simulink model "V2G_FDCC"  (R2024a)
settings: Solver=FixedStepAuto  StartTime=0.0  StopTime=10  FixedStep=1e-5  MaxStep=1.0E-5  RelTol=1e-3
values from neighbouring files (symbols this model uses):
  Batt_Ah = 2000    [main_v2gg2v.m]
  Batt_RespTime = 1    [main_v2gg2v.m]
  Batt_Vnom = 800    [main_v2gg2v.m]
  C_inv = (r*(Pinv/3)*al*(-be+al-1))/(100*Vac_l_rms*Vin_inv*wn*(al-be))    [main_v2gg2v.m]    (also in script.m = 0.00198943678865)
  C_mppt = 20*(Iout_mppt*D_mppt)/(deltaV*fs_mppt)    (= 0.0948148148148)    [main_v2gg2v.m]    (also in script.m)
  C_Vdc = 100*18e-3    (= 1.8)    [main_v2gg2v.m]
  cap_bat = 2000    [main_v2gg2v.m]    (also in script.m)
  Cbat_buck = deltaI_bat/(8*fs_bat*deltaV_bat)    (= 0.00133333333333)    [main_v2gg2v.m]    (also in script.m)
  Cdc = 30e-3    (= 0.03)    [main_v2gg2v.m]    (also in script.m)
  Cdc_boost = 50*Cbat_buck    (= 0.0666666666667)    [main_v2gg2v.m]    (also in script.m)
  Cf = 10*165e-6    (= 0.00165)    [main_v2gg2v.m]
  D = 2    [main_v2gg2v.m]
  Dinv = 0    [main_v2gg2v.m]
  f_grid = 50    [main_v2gg2v.m]
  fg = 50    [main_v2gg2v.m]    (also in script.m)
  H1 = 7    [main_v2gg2v.m]
  H2 = 8    [main_v2gg2v.m]
  H3 = 12    [main_v2gg2v.m]
  Hinv = 0    [main_v2gg2v.m]
  Ki_CC = 1    [main_v2gg2v.m]
  Ki_inner = 5000    [main_v2gg2v.m]
  Ki_outer = 10000    [main_v2gg2v.m]
  Ki_PLL = 10000    [main_v2gg2v.m]
  Kp_CC = 10    [main_v2gg2v.m]
  Kp_inner = 100    [main_v2gg2v.m]
  Kp_outer = 250    [main_v2gg2v.m]
  Kp_PLL = 100    [main_v2gg2v.m]
  L_bat = (Vbat*(Vdc_link-Vbat))/(deltaI_bat*fs_bat*Vdc_link)    (= 0.001875)    [main_v2gg2v.m]    (also in script.m)
  L_mppt = 1*(Vpv*D_mppt)/(deltaI*fs_mppt)    (= 0.000161333333333)    [main_v2gg2v.m]    (also in script.m)
  Lgrid = 1/10*0.69e-3    (= 6.9e-05)    [main_v2gg2v.m]
  Linv = 1/10*0.48e-3    (= 4.8e-05)    [main_v2gg2v.m]
  Lmin_inv = (100*Vac_l_rms*Vin_inv*(al-be))/(wn*r*(Pinv/3)*(-be+al-1))    [main_v2gg2v.m]    (also in script.m = 0.000611154981473)
  LowSat_CC = 0    [main_v2gg2v.m]
  omega = 2*pi*f_grid    (= 314.159265359)    [main_v2gg2v.m]
  Pinv = 2e6    (= 2000000)    [main_v2gg2v.m]    (also in script.m)
  Rd = 1.31    [main_v2gg2v.m]
  Sbase = 1e6    (= 1000000)    [main_v2gg2v.m]    (also in script.m)
  Snom_trafo = 1050e6    (= 1050000000)    [main_v2gg2v.m]
  t_fault_end = t_fault_start + FCT    (= 1.1)    [main_v2gg2v.m]
  t_fault_start = 1    [main_v2gg2v.m]
  Ts = 1e-5    (= 1e-05)    [main_v2gg2v.m]
  UpSat_CC = 1    [main_v2gg2v.m]
  Vac_inv = 800    [main_v2gg2v.m]    (also in script.m)
  Vbase = 345e3    (= 345000)    [main_v2gg2v.m]    (also in script.m)
  Vbat = 750    [main_v2gg2v.m]    (also in script.m)
  Vdc_ref = 1.5e3    (= 1500)    [main_v2gg2v.m]
  wg = 2*pi*fg    (= 314.159265359)    [main_v2gg2v.m]    (also in script.m)
undefined symbols (not defined in the file or in its folder): Acid, D1, Delta, h_PEV, Ibatfault_ref, ibatref, Ion, L12, L13, L23, Lbat, Lbuckboost, Lead, Lithium, R_Vdc, Rbuckboost, Vfault_thresh, vthref
libraries: spsSeriesRLCBranchLib x74, slpidlib x62, spsMosfetLib x50, spsGroundLib x48, spsBatteryLib x31, eeGeneralControl x31, spsPWMGeneratorDCDCLib x29, spsCurrentMeasurementLib x28, spsThreePhaseSeriesRLCBranchLib x21, spsThreePhaseVIMeasurementLib x18, spsIGBTDiodeLib x18, spsVoltageMeasurementLib x14
(part 1 of 11)
settings Model: Creator=BagaskaraPP  LastModifiedBy=hp
settings SolverCC: ZeroCrossAlgorithm=Adaptive  AlgebraicLoopSolver=TrustRegion
settings DataIOCC: ExternalInput=getinputstruct(op1)  InitialState=getstatestruct(op1)  SaveFormat=StructureWithTime  SaveOutput=off  ReturnWorkspaceOutputs=off  Refine=4
settings DebuggingCC: AlgebraicLoopMsg=none  MaxConsecutiveZCsMsg=none  IgnoredZcDiagnostic=none  ArithmeticOperatorsInVariantConditions=warning
settings ModelReferenceCC: EnableRefExpFcnMdlSchedulingChecks=on
settings SFSimCC: SimUseLocalCustomCode=off  CustomCodeUndefinedFunction=UseInterfaceOnly
settings RTWCC: RTWUseLocalCustomCode=off  GPUComputeCapability=3.5
settings CodeAppCC: StateflowObjectComments=on
settings SimscapeCC: SimscapeNormalizeSystem=off

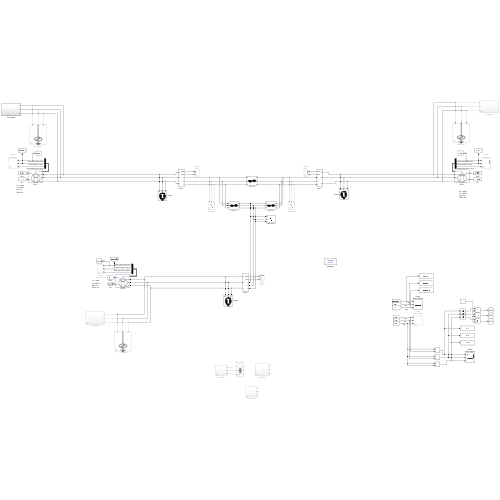
[thumbnail: Simulink's stored preview of the top-level diagram]
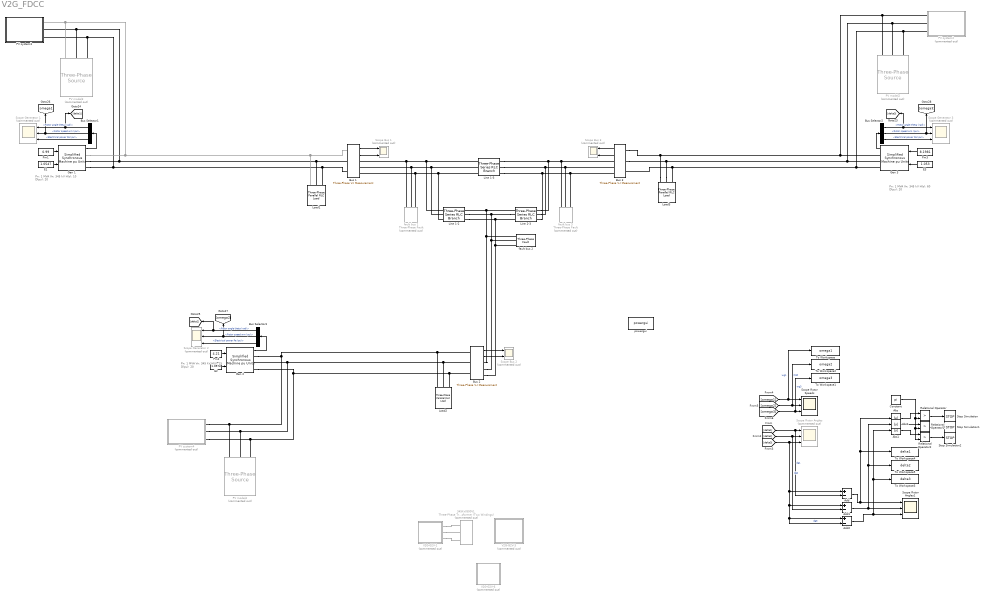
== system V2G_FDCC ==
  note: Pn: 1 MVA
      | Vn: 345 kV
      | H(s): 15
      | D(pu): 20
  note: Pn: 1 MVA
      | Vn: 345 kV
      | H(s): 60
      | D(pu): 20
  note: Pn: 1 MVA
      | Vn: 345 kV
      | H(s): 10
      | D(pu): 20
  345kV/800V1 : spsThreePhaseTransformerTwoWindingsLib/Three-Phase Transformer (Two Windings)  Commented=on  Winding1Connection=Delta (D1)  Winding2Connection=Yg  CoreType=Three single-phase transformers  SetSaturation=off  Hysteresis=off  DataFile='hysteresis'  SetInitialFlux=off  Measurements=None  UNITS=pu  NominalPower=[ Snom_trafo , f_grid ]  Winding1=[Vbase , 0 , 0 ]  Winding2=[ 800 , 0 , 0 ]  Rm=0  Lm=0  L0=0.5  Saturation=[ 0,0 ; 0.0024,1.2 ; 1.0,1.52 ]  InitialFluxes=[ 0.8 , -0.8 , 0.7 ]  BreakLoop=off  DiscreteSolver=Trapezoidal iterative  DataType=off  TransfoNumber=1
  Abs : Abs  SaturateOnIntegerOverflow=off
  Abs1 : Abs  SaturateOnIntegerOverflow=off
  Abs2 : Abs  SaturateOnIntegerOverflow=off
  Add : Sum  Inputs=+-
  Add1 : Sum  Inputs=+-
  Add2 : Sum  Inputs=+-
  Bus Selector1 : BusSelector  OutputSignals=Rotor angle theta (rad),Rotor speed wm (pu),Electrical power Pe (pu)
  Bus Selector2 : BusSelector  OutputSignals=Rotor angle theta (rad),Rotor speed wm (pu),Electrical power Pe (pu)
  Bus Selector3 : BusSelector  OutputSignals=Rotor angle theta (rad),Rotor speed wm (pu),Electrical power Pe (pu)
  Bus 1 : spsThreePhaseVIMeasurementLib/Three-Phase V-I Measurement  VoltageMeasurement=phase-to-ground  SetLabelV=off  LabelV=Vabc  Vpu=off  VpuLL=off  CurrentMeasurement=yes  SetLabelI=off  LabelI=Iabc  Ipu=off  Pbase=100e6  Vbase=500e3  OutputType=Complex  PhasorSimulation=off  PSBequivalent=0
  Bus 2 : spsThreePhaseVIMeasurementLib/Three-Phase V-I Measurement  VoltageMeasurement=phase-to-ground  SetLabelV=off  LabelV=Vabc  Vpu=off  VpuLL=off  CurrentMeasurement=yes  SetLabelI=off  LabelI=Iabc  Ipu=off  Pbase=100e6  Vbase=500e3  OutputType=Complex  PhasorSimulation=off  PSBequivalent=0
  Bus 3 : spsThreePhaseVIMeasurementLib/Three-Phase V-I Measurement  VoltageMeasurement=phase-to-ground  SetLabelV=off  LabelV=Vabc  Vpu=off  VpuLL=off  CurrentMeasurement=yes  SetLabelI=off  LabelI=Iabc  Ipu=off  Pbase=100e6  Vbase=500e3  OutputType=Complex  PhasorSimulation=off  PSBequivalent=0
  Constant : Constant  Value=pi
  E1 : Constant  Value=1.0547
  E2 : Constant  Value=1.0573
  E3 : Constant  Value=1.053
  Gen 1 : spsSimplifiedSynchronousMachinepuUnitsLib/Simplified Synchronous Machine pu Units  ConnectionType=3-wire Y  MechanicalLoad=Mechanical power Pm  MeasurementBus=off  NominalParameters=[Sbase Vbase f_grid]  Mechanical=[H1 D 1]  InternalRL="[0.0  0.088]"  InitialConditions=[0 19.7482 1.15593 1.15593 1.15593 -15.1433 -135.143 104.857]  IterativeDiscreteModel=Trapezoidal non iterative  TsBlock=-1  TsPowergui=0  LoadFlowParameters=[1,0,0,0,0]  Units=0  BusType=PV  Pref=1000000  Qref=0  Qmin=-Inf  Qmax=Inf  PLF=0  QLF=0
      settings: LibrarySourceBlock=|
      | sps_lib/Electrical Machines/Simplified Synchronous
      | Machine pu Units
  Gen 2 : spsSimplifiedSynchronousMachinepuUnitsLib/Simplified Synchronous Machine pu Units  ConnectionType=3-wire Y  MechanicalLoad=Mechanical power Pm  MeasurementBus=off  NominalParameters=[Sbase Vbase f_grid]  Mechanical=[H2 D 1]  InternalRL="[0.0  0.05]"  InitialConditions=[0 26.4733 4.27149 4.27149 4.27149 5.25563 -114.744 125.256]  IterativeDiscreteModel=Trapezoidal non iterative  TsBlock=-1  TsPowergui=0  LoadFlowParameters=[1,0,0,0,0]  Units=0  BusType=PV  Pref=4210000  Qref=0  Qmin=-Inf  Qmax=Inf  PLF=0  QLF=0
      settings: LibrarySourceBlock=|
      | sps_lib/Electrical Machines/Simplified Synchronous
      | Machine pu Units
  Gen 3 : spsSimplifiedSynchronousMachinepuUnitsLib/Simplified Synchronous Machine pu Units  ConnectionType=3-wire Y  MechanicalLoad=Mechanical power Pm  MeasurementBus=off  NominalParameters=[Sbase Vbase f_grid]  Mechanical=[H3 D 1]  InternalRL="[0.0  0.015]"  InitialConditions=[0 6.70648 8.74798 8.74798 8.74798 -20.4227 -140.423 99.5773]  IterativeDiscreteModel=Trapezoidal non iterative  TsBlock=-1  TsPowergui=0  LoadFlowParameters=[1,0,0,0,0]  Units=0  BusType=swing  Pref=6200000  Qref=0  Qmin=-Inf  Qmax=Inf  PLF=0  QLF=0
      settings: LibrarySourceBlock=|
      | sps_lib/Electrical Machines/Simplified Synchronous
      | Machine pu Units
  Line 1-2 : spsThreePhaseSeriesRLCBranchLib/Three-Phase Series RLC Branch  LConnTagsString=A|B|C  RConnTagsString=A|B|C  BranchType=RL  Resistance=0  Inductance=L12  Capacitance=1e-6  Measurements=None
  Line 1-3 : spsThreePhaseSeriesRLCBranchLib/Three-Phase Series RLC Branch  LConnTagsString=A|B|C  RConnTagsString=A|B|C  BranchType=RL  Resistance=0  Inductance=L13  Capacitance=1e-6  Measurements=None
  Line 2-3 : spsThreePhaseSeriesRLCBranchLib/Three-Phase Series RLC Branch  LConnTagsString=A|B|C  RConnTagsString=A|B|C  BranchType=RL  Resistance=0  Inductance=L23  Capacitance=1e-6  Measurements=None
  Load1 : spsThreePhaseParallelRLCLoadLib/Three-Phase Parallel RLC Load  LConnTagsString=A|B|C  Configuration=Y (grounded)  NominalVoltage=(345000)*1  Vabc=[1e3 1e3 1e3]  Vabcp=[1e3 1e3 1e3]  NominalFrequency=f_grid  UnbalancedPower=off  ActivePower=1500000  InductivePower=450000  CapacitivePower=0  Pabc=[10e3 9e3 11e3]  QLabc=[100 90 110]  QCabc=[100 90 110]  Pabcp=[10e3 9e3 11e3]  QLabcp=[100 90 110]  QCabcp=[100 90 110]  Measurements=None  LoadType=constant PQ
  Load2 : spsThreePhaseParallelRLCLoadLib/Three-Phase Parallel RLC Load  LConnTagsString=A|B|C  Configuration=Y (grounded)  NominalVoltage=(345000)*1  Vabc=[1e3 1e3 1e3]  Vabcp=[1e3 1e3 1e3]  NominalFrequency=f_grid  UnbalancedPower=off  ActivePower=1000000  InductivePower=300000  CapacitivePower=0  Pabc=[10e3 9e3 11e3]  QLabc=[100 90 110]  QCabc=[100 90 110]  Pabcp=[10e3 9e3 11e3]  QLabcp=[100 90 110]  QCabcp=[100 90 110]  Measurements=None  LoadType=constant PQ
  Load3 : spsThreePhaseParallelRLCLoadLib/Three-Phase Parallel RLC Load  LConnTagsString=A|B|C  Configuration=Y (grounded)  NominalVoltage=(345000)*1  Vabc=[1e3 1e3 1e3]  Vabcp=[1e3 1e3 1e3]  NominalFrequency=f_grid  UnbalancedPower=off  ActivePower=12400000  InductivePower=2500000  CapacitivePower=0  Pabc=[10e3 9e3 11e3]  QLabc=[100 90 110]  QCabc=[100 90 110]  Pabcp=[10e3 9e3 11e3]  QLabcp=[100 90 110]  QCabcp=[100 90 110]  Measurements=None  LoadType=constant PQ
  PV model2 : spsThreePhaseSourceLib/Three-Phase Source  Commented=on  InternalConnection=Yg  VoltagePhases=off  Voltage=(345000)*1  PhaseAngle=0  Voltage_phases=[25e3 25e3 25e3]/sqrt(3)  PhaseAngles_phases=[0 -120 +120]  Frequency=fg  NonIdealSource=off  SpecifyImpedance=off  Resistance=0.8929  Inductance=16.58e-3  ShortCircuitLevel=100e6  BaseVoltage=25e3  XRratio=7  BusType=PQ  Pref=1492000  Qref=606.9  Prefabc=[10e3, 10e3, 10e3]  Qrefabc=[0, 0, 0]  Qmin=-Inf  Qmax=Inf
  PV model3 : spsThreePhaseSourceLib/Three-Phase Source  Commented=on  InternalConnection=Yg  VoltagePhases=off  Voltage=(345000)*1  PhaseAngle=14.9621  Voltage_phases=[25e3 25e3 25e3]/sqrt(3)  PhaseAngles_phases=[0 -120 +120]  Frequency=fg  NonIdealSource=off  SpecifyImpedance=off  Resistance=0.8929  Inductance=16.58e-3  ShortCircuitLevel=100e6  BaseVoltage=25e3  XRratio=7  BusType=PQ  Pref=1492000  Qref=606.9  Prefabc=[10e3, 10e3, 10e3]  Qrefabc=[0, 0, 0]  Qmin=-Inf  Qmax=Inf
  PV model4 : spsThreePhaseSourceLib/Three-Phase Source  Commented=on  InternalConnection=Yg  VoltagePhases=off  Voltage=(345000)*1  PhaseAngle=21.4896  Voltage_phases=[25e3 25e3 25e3]/sqrt(3)  PhaseAngles_phases=[0 -120 +120]  Frequency=fg  NonIdealSource=off  SpecifyImpedance=off  Resistance=0.8929  Inductance=16.58e-3  ShortCircuitLevel=100e6  BaseVoltage=25e3  XRratio=7  BusType=PQ  Pref=1492000  Qref=606.9  Prefabc=[10e3, 10e3, 10e3]  Qrefabc=[0, 0, 0]  Qmin=-Inf  Qmax=Inf
  PV system2 : Subsystem  Commented=on
  PV system3 : Subsystem
  PV system4 : Subsystem  Commented=on
  Pm1 : Constant  Value=0.99
  Pm2 : Constant  Value=4.21
  Pm3 : Constant  Value=8.1981
  Relational Operator : RelationalOperator  Operator=>  OutDataTypeStr=boolean  RndMeth=Simplest  InputSameDT=off
  Relational Operator1 : RelationalOperator  Operator=>  OutDataTypeStr=boolean  RndMeth=Simplest  InputSameDT=off
  Relational Operator2 : RelationalOperator  Operator=>  OutDataTypeStr=boolean  RndMeth=Simplest  InputSameDT=off
  Scope Bus 1 : Scope  Commented=on  NumInputPorts=2
  Scope Bus 2 : Scope  Commented=on  NumInputPorts=2
  Scope Bus 3 : Scope  Commented=on  NumInputPorts=2
  Scope Generator 1 : Scope  Commented=on  NumInputPorts=3
  Scope Generator 2 : Scope  Commented=on  NumInputPorts=3
  Scope Generator 3 : Scope  Commented=on  NumInputPorts=3
  Scope Rotor Angles : Scope  Commented=on  NumInputPorts=3
  Scope Rotor Angles1 : Scope  NumInputPorts=3
  Scope Rotor Speeds : Scope  NumInputPorts=3
  Stop Simulation : Stop
  Stop Simulation1 : Stop
  Stop Simulation2 : Stop
  To Workspace : ToWorkspace  VariableName=omega1  SaveFormat=Timeseries  SampleTime=-1
  To Workspace1 : ToWorkspace  VariableName=omega3  SaveFormat=Timeseries  SampleTime=-1
  To Workspace2 : ToWorkspace  VariableName=omega2  SaveFormat=Timeseries  SampleTime=-1
  To Workspace3 : ToWorkspace  VariableName=delta3  SaveFormat=Timeseries  SampleTime=-1
  To Workspace4 : ToWorkspace  VariableName=delta1  SaveFormat=Timeseries  SampleTime=-1
  To Workspace5 : ToWorkspace  VariableName=delta2  SaveFormat=Timeseries  SampleTime=-1
  V2G-G2V-1 : Subsystem  Commented=on
  V2G-G2V-3 : Subsystem  Commented=on
  V2G-G2V-6 : Subsystem  Commented=on
  fault bus 1 : spsThreePhaseFaultLib/Three-Phase Fault  Commented=on  InitialStates=0  FaultA=on  FaultB=on  FaultC=on  GroundFault=off  SwitchTimes="[t_fault_start  t_fault_end]"  External=off  SwitchStatus=NaN  FaultResistance=0.001  GroundResistance=0.01  SnubberResistance=1e6  SnubberCapacitance=inf  Measurements=None
  fault bus 2 : spsThreePhaseFaultLib/Three-Phase Fault  InitialStates=0  FaultA=on  FaultB=on  FaultC=on  GroundFault=off  SwitchTimes="[t_fault_start  t_fault_end]"  External=off  SwitchStatus=NaN  FaultResistance=0.001  GroundResistance=0.01  SnubberResistance=1e6  SnubberCapacitance=inf  Measurements=None
  fault bus 3 : spsThreePhaseFaultLib/Three-Phase Fault  Commented=on  InitialStates=0  FaultA=on  FaultB=on  FaultC=on  GroundFault=off  SwitchTimes="[t_fault_start  t_fault_end]"  External=off  SwitchStatus=NaN  FaultResistance=0.001  GroundResistance=0.01  SnubberResistance=1e6  SnubberCapacitance=inf  Measurements=None
  powergui : sps_lib/powergui  Priority=1  SimulationMode=Discrete  SampleTime=1e-5  frequency=60  Iterations=200  frequencyindice=50  Pbase=1e6  ErrMax=1e-4  UnitsV=kV  UnitsW=MW  buscounter=1  FunctionMessages=off  echomessages=off  EnableUseOfTLC=off  CurrentSourceSwitches=off  DisableSnubberDevices=off  DisableRonSwitches=off  DisableVfSwitches=off  DisplayEquations=off  AutomaticDiscreteSolvers=off  SolverType=Tustin/Backward Euler (TBE)  Interpol=off  ExternalGateDelay=off  methode=off  Ts=100  x0status=blocks  SPID=on  SwTol=0  HookPort=off  NonlinearTolerance=1e-4  nMaxIteration=100  ContinueOnMaxIteration=off  RestoreLinks=warning  ResistiveCurrentMeasurement=off  Frange=[0:2:500]  Ylog=off  Xlog=on  ShowGrid=off  save=off  variable=ZData  structure=0  ZoomFFT=off  StartTime=0.0  cycles=1  DisplayStyle=1  fundamental=60  FreqAxis=off  MaxFrequency=1000  frequencyindicesteady=1  RmsSteady=1  display=off
  wires:
  Bus 1/1 -> Scope Bus 1/1
  Pm2/1 -> Gen 2/1
  Bus Selector2/2 -> [omega3], Scope Generator 3/2  "<Rotor speed wm (pu)>"
  Bus Selector2/1 -> Scope Generator 3/1, [delta3]  "<Rotor angle theta (rad)>"
  Pm3/1 -> Gen 3/1
  Bus 2/2 -> Scope Bus 2/2
  Bus Selector3/3 -> Scope Generator 2/3  "<Electrical power Pe (pu)>"
  Bus Selector2/3 -> Scope Generator 3/3  "<Electrical power Pe (pu)>"
  Bus 1/2 -> Scope Bus 1/2
  Bus Selector3/2 -> Scope Generator 2/2, [omega2]  "<Rotor speed wm (pu)>"
  Bus 3/2 -> Scope Bus 3/2
  Bus Selector3/1 -> Scope Generator 2/1, [delta2]  "<Rotor angle theta (rad)>"
  Bus 3/1 -> Scope Bus 3/1
  Bus 2/1 -> Scope Bus 2/1
  E1/1 -> Gen 1/2
  Pm1/1 -> Gen 1/1
  Gen 1/1 -> Bus Selector1/1
  Bus Selector1/3 -> Scope Generator 1/3  "<Electrical power Pe (pu)>"
  Gen 3/1 -> Bus Selector2/1
  Bus Selector1/2 -> Scope Generator 1/2, [omega1]  "<Rotor speed wm (pu)>"
  Bus Selector1/1 -> Scope Generator 1/1, [delta1]  "<Rotor angle theta (rad)>"
  Gen 2/1 -> Bus Selector3/1
  E2/1 -> Gen 2/2
  E3/1 -> Gen 3/2
  [omega2] -> To Workspace2/1, Scope Rotor Speeds/2  "wg2"
  [delta2] -> Add1/2, Scope Rotor Angles/2  "dg2"
  [delta3] -> Add/1, Add1/1, Add2/2, Add2/1, Scope Rotor Angles/3  "dg3"
  [delta1] -> Add/2, Scope Rotor Angles/1  "dg1"
  [omega3] -> To Workspace1/1, Scope Rotor Speeds/3  "wg3"
  [omega1] -> To Workspace/1, Scope Rotor Speeds/1  "wg1"
  Add1/1 -> Abs2/1, To Workspace5/1, Scope Rotor Angles1/2
  Add/1 -> Abs/1, To Workspace4/1, Scope Rotor Angles1/1
  Add2/1 -> Abs1/1, To Workspace3/1, Scope Rotor Angles1/3
  Abs/1 -> Relational Operator/1
  Abs2/1 -> Relational Operator1/1
  Abs1/1 -> Relational Operator2/1
  Relational Operator/1 -> Stop Simulation/1
  Constant/1 -> Relational Operator2/2, Relational Operator1/2, Relational Operator/2
  Relational Operator2/1 -> Stop Simulation2/1
  Relational Operator1/1 -> Stop Simulation1/1
  connections:
  Line 1-2/LConn1 -- Line 1-3/LConn1 -- fault bus 1/LConn1 -- Bus 1/RConn1
  Load1/LConn3 -- PV model3/RConn3 -- PV system3/RConn3 -- Gen 1/RConn3 -- Bus 1/LConn3
  Line 2-3/LConn2 -- Bus 2/RConn2 -- fault bus 2/LConn2 -- Line 1-2/RConn2
  Gen 3/RConn3 -- Bus 3/LConn3 -- Load3/LConn3 -- PV model2/RConn3 -- PV system2/RConn3
  Bus 3/RConn2 -- fault bus 3/LConn2 -- Line 2-3/RConn2 -- Line 1-3/RConn2
  Bus 3/RConn3 -- fault bus 3/LConn3 -- Line 2-3/RConn3 -- Line 1-3/RConn3
  PV system3/RConn2 -- PV model3/RConn2 -- Load1/LConn2 -- Bus 1/LConn2 -- Gen 1/RConn2
  Load3/LConn1 -- PV model2/RConn1 -- PV system2/RConn1 -- Gen 3/RConn1 -- Bus 3/LConn1
  Line 2-3/LConn1 -- Bus 2/RConn1 -- fault bus 2/LConn1 -- Line 1-2/RConn1
  Load3/LConn2 -- PV model2/RConn2 -- PV system2/RConn2 -- Gen 3/RConn2 -- Bus 3/LConn2
  Line 1-3/RConn1 -- Bus 3/RConn1 -- fault bus 3/LConn1 -- Line 2-3/RConn1
  Line 1-3/LConn2 -- Line 1-2/LConn2 -- fault bus 1/LConn2 -- Bus 1/RConn2
  Line 1-2/LConn3 -- Line 1-3/LConn3 -- fault bus 1/LConn3 -- Bus 1/RConn3
  PV model3/RConn1 -- PV system3/RConn1 -- Load1/LConn1 -- Bus 1/LConn1 -- Gen 1/RConn1
  Bus 2/RConn3 -- fault bus 2/LConn3 -- Line 2-3/LConn3 -- Line 1-2/RConn3
  V2G-G2V-1/LConn1 -- 345kV/800V1/RConn1
  V2G-G2V-1/LConn2 -- 345kV/800V1/RConn2
  V2G-G2V-1/LConn3 -- 345kV/800V1/RConn3
  Gen 2/RConn1 -- Load2/LConn1 -- Bus 2/LConn1 -- PV model4/RConn1 -- PV system4/RConn1
  Load2/LConn2 -- PV model4/RConn2 -- PV system4/RConn2 -- Gen 2/RConn2 -- Bus 2/LConn2
  Gen 2/RConn3 -- PV model4/RConn3 -- PV system4/RConn3 -- Bus 2/LConn3 -- Load2/LConn3

== system V2G_FDCC/PV system2 ==
  note: P = 1.96e6
      | Q = -0.6842
  Battery1 : spsBatteryLib/Battery  BatType=Lead-Acid  ShowTempParam=off  ThermalPreset="12.8V  40Ah  (LiFeMgPO4)"  ShowAgeParam=off  NomV=Vbat  NomQ=cap_bat  SOC=50  Batt_Tr=2  PresetModel=off  MaxQ=cap_bat  MinV=0.8*Vbat  FullV=1.1*Vbat  Dis_rate=Inom_bat  R=0.002  Normal_OP=0.9*cap_bat  expZone="[780   20]"  current=[250 500 750 1000]  Units=Ampere-hour  Tci=20  NomT=20  T2=-30  MaxQ2=4.8  FullV2=7.1  Normal_OP2=5.655  expZone2="[6.58           1]"  Rca=0.6  ti=2000  Dp=0  Neq0=0  Tsim=1e6  Ta1=25  Qeol=5.4*0.9  Reol=0.013333*1.2  Char_age=[2.3478, 3]  Dis_age=[2.3478, 10]  N1=1500  N2=10500  N3=1000  N4=1400  Ta2=45  N5=950
  Bus x : spsThreePhaseVIMeasurementLib/Three-Phase V-I Measurement  VoltageMeasurement=phase-to-ground  SetLabelV=off  LabelV=Vabc  Vpu=off  VpuLL=off  CurrentMeasurement=yes  SetLabelI=off  LabelI=Iabc  Ipu=off  Pbase=100e6  Vbase=13.8e3  OutputType=Complex  PhasorSimulation=off  PSBequivalent=0
  Cdc link1 : spsSeriesRLCBranchLib/Series RLC Branch  LConnTagsString=__new0  RConnTagsString=__new0  BranchType=C  Resistance=0.001  Inductance=1e-3  SetiL0=off  InitialCurrent=0  Capacitance=Cdc  Setx0=on  InitialVoltage=1500  Measurements=None
  Current Measurement1 : spsCurrentMeasurementLib/Current Measurement  PhasorSimulation=off  OutputType=Complex  PSBequivalent=0
  Current Measurement3 : spsCurrentMeasurementLib/Current Measurement  PhasorSimulation=off  OutputType=Complex  PSBequivalent=0
  DC-DC Converter Bidirectional1 : Subsystem
  DC-DC Converter Unidirectional1 : Subsystem
  Ground{2,9,12,14} (4 alike) : spsGroundLib/Ground  LConnTagsString=a
  Inverter : Subsystem
  Irradiance1 : Constant  Value=1000
  Ldc1 : spsSeriesRLCBranchLib/Series RLC Branch  LConnTagsString=__new0  RConnTagsString=__new0  BranchType=L  Resistance=0.002  Inductance=10e-3  SetiL0=off  InitialCurrent=0  Capacitance=5e-3  Setx0=on  InitialVoltage=0  Measurements=None
  Low-Pass Filter (Discrete or Continuous) : eeGeneralControl/Low-Pass Filter (Discrete or Continuous)  Commented=on  K=1  T=1/(2*pi*5)  B=inf  A=-inf  init_option=Inherited from block input  x0=0  Ts=-1
  Low-Pass Filter (Discrete or Continuous)2 : eeGeneralControl/Low-Pass Filter (Discrete or Continuous)  Commented=on  K=1  T=1/(2*pi*5)  B=inf  A=-inf  init_option=Inherited from block input  x0=0  Ts=-1
  PV Solar Array1 : spsPVArrayLib/PV Array  Npar=278  Nser=15  PlotType=array @ 1000 W/m2 & specified temperatures  S_vec=[ 1000 800 500 300 100 ]  Temp_C_vec=[ 20 25 30 35 ]  ModuleName=Sunpower SPR-X22-480-COM  PlotWhenSelected=off  Pm=480.32  Ncell=128  Voc=92.9  Isc=6.48  Vm=79  Im=6.08  beta_Voc_pc=-0.293  alpha_Isc_pc=0.031003  beta_Voc=-0.2722  alpha_Isc=0.002009  IL=6.4884  I0=1.5908e-11  nI=1.0576  Rsh=598.2816  Rs=0.48607  RobustModel=off  RobustCellTemperature=313.3991  BAL=on  Tc=1e-6  Tfilter=5e-5
  PV model2 : spsThreePhaseSourceLib/Three-Phase Source  Commented=on  InternalConnection=Yg  VoltagePhases=off  Voltage=(345000)*1  PhaseAngle=0  Voltage_phases=[25e3 25e3 25e3]/sqrt(3)  PhaseAngles_phases=[0 -120 +120]  Frequency=fg  NonIdealSource=off  SpecifyImpedance=off  Resistance=0.8929  Inductance=16.58e-3  ShortCircuitLevel=100e6  BaseVoltage=25e3  XRratio=7  BusType=swing  Pref=1993000  Qref=10680  Prefabc=[10e3, 10e3, 10e3]  Qrefabc=[0, 0, 0]  Qmin=-Inf  Qmax=Inf
  Power (Positive-Sequence) : spsPowerPositiveSequenceLib/Power (Positive-Sequence)  Commented=on  Freq=50  Vinit=[0, 0]  Iinit=[0, 0]  Ts=1e-5
      settings: LibrarySourceBlock=|
      | sps_lib/Sensors and Measurements/Power
      | (Positive-Sequence)
  Product : Product  Commented=on
  Scope3 : Scope  Commented=on  NumInputPorts=2
  Scope5 : Scope  Commented=on  NumInputPorts=2
  Scope9 : Scope  Commented=on  NumInputPorts=3
  Temp1 : Constant  Value=25
  Three-Phase Transformer : spsThreePhaseTransformerTwoWindingsLib/Three-Phase Transformer (Two Windings)  Winding1Connection=Yg  Winding2Connection=Delta (D1)  CoreType=Three single-phase transformers  SetSaturation=off  Hysteresis=off  DataFile='hysteresis'  SetInitialFlux=off  Measurements=None  UNITS=pu  NominalPower=[ Pinv*2 , fg ]  Winding1=[Vbase 1e-6 1e-6]  Winding2=[Vac_inv 1e-6 1e-6]  Rm=500  Lm=1000  L0=0.5  Saturation=[0 0;0.01 0.9;0.05 1]  InitialFluxes=[-1.0025142026259 0.501432695325379 0.501081507300505]  BreakLoop=off  DiscreteSolver=Trapezoidal iterative  DataType=off  TransfoNumber=1
  Voltage Measurement1 : spsVoltageMeasurementLib/Voltage Measurement  PhasorSimulation=off  OutputType=Complex  PSBequivalent=0
  Voltage Measurement2 : spsVoltageMeasurementLib/Voltage Measurement  PhasorSimulation=off  OutputType=Complex  PSBequivalent=0
  a : PMIOPort  Side=Right
  b : PMIOPort  Port=2  Side=Right
  c : PMIOPort  Port=3  Side=Right
  wires:
  Voltage Measurement2/1 -> Scope5/1  "Vout"
  Irradiance1/1 -> PV Solar Array1/1
  Low-Pass Filter (Discrete or Continuous)/1 -> Scope3/1  "Pout"
  Power (Positive-Sequence)/1 -> Low-Pass Filter (Discrete or Continuous)/1
  Current Measurement1/1 -> Scope5/2  "iout"
  Voltage Measurement1/1 -> [Vdc], Product/1, Scope9/1
  Current Measurement3/1 -> Product/2, Scope9/2
  Low-Pass Filter (Discrete or Continuous)2/1 -> Scope3/2  "Qout"
  [Vdc] -> DC-DC Converter Bidirectional1/1(Vdclink)
  Bus x/2 -> Power (Positive-Sequence)/2
  Temp1/1 -> PV Solar Array1/2
  Bus x/1 -> Power (Positive-Sequence)/1
  Power (Positive-Sequence)/2 -> Low-Pass Filter (Discrete or Continuous)2/1
  Product/1 -> Scope9/3
  connections:
  Inverter/RConn1 -- Current Measurement1/LConn1
  PV Solar Array1/RConn1 -- DC-DC Converter Unidirectional1/LConn1
  Voltage Measurement2/LConn1 -- Current Measurement1/RConn1 -- Three-Phase Transformer/RConn1
  Voltage Measurement2/LConn2 -- Inverter/RConn2 -- Three-Phase Transformer/RConn2
  Inverter/LConn1 -- Voltage Measurement1/LConn1 -- Current Measurement3/RConn1
  Three-Phase Transformer/RConn3 -- Inverter/RConn3
  Battery1/LConn2 -- Ground2/LConn1
  Three-Phase Transformer/LConn3 -- Bus x/LConn3
  Voltage Measurement1/LConn2 -- Ground9/LConn1
  PV Solar Array1/RConn2 -- Ground14/LConn1
  Battery1/LConn1 -- DC-DC Converter Bidirectional1/LConn1
  Ground12/LConn1 -- Cdc link1/RConn1
  Three-Phase Transformer/LConn1 -- Bus x/LConn1
  Current Measurement3/LConn1 -- Cdc link1/LConn1 -- DC-DC Converter Bidirectional1/RConn1 -- Ldc1/RConn1
  Three-Phase Transformer/LConn2 -- Bus x/LConn2
  Ldc1/LConn1 -- DC-DC Converter Unidirectional1/RConn1
  Bus x/RConn2 -- b/RConn1 -- PV model2/RConn2
  Bus x/RConn1 -- a/RConn1 -- PV model2/RConn1
  Bus x/RConn3 -- c/RConn1 -- PV model2/RConn3

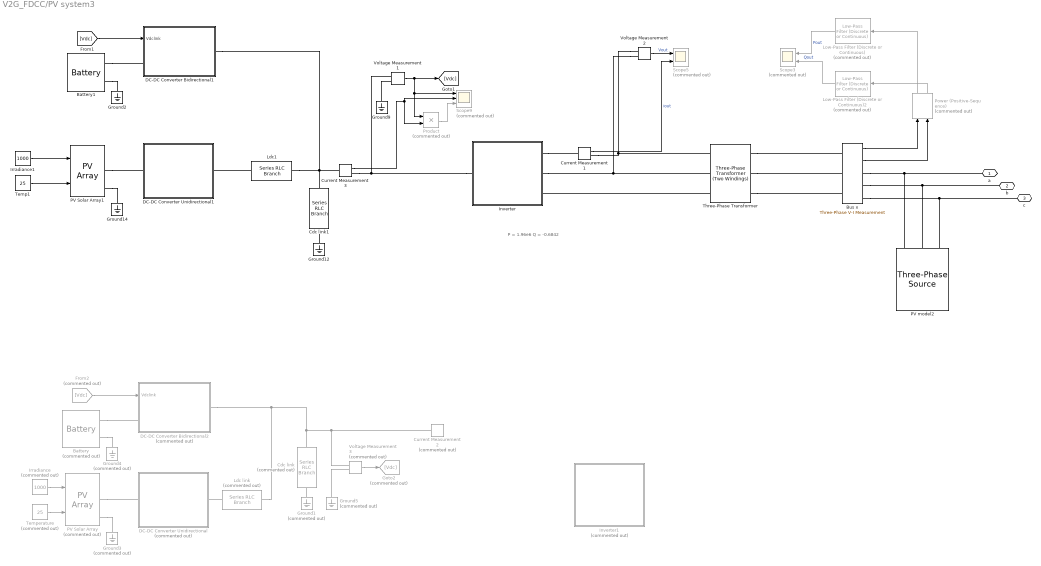
== system V2G_FDCC/PV system3 ==
  note: P = 1.96e6
      | Q = -0.6842
  Battery : spsBatteryLib/Battery  Commented=on  BatType=Lead-Acid  ShowTempParam=off  ThermalPreset="12.8V  40Ah  (LiFeMgPO4)"  ShowAgeParam=off  NomV=Vbat  NomQ=cap_bat  SOC=50  Batt_Tr=2  PresetModel=off  MaxQ=cap_bat  MinV=0.8*Vbat  FullV=1.1*Vbat  Dis_rate=Inom_bat  R=0.002  Normal_OP=0.9*cap_bat  expZone="[780   20]"  current=[250 500 750 1000]  Units=Ampere-hour  Tci=20  NomT=20  T2=-30  MaxQ2=4.8  FullV2=7.1  Normal_OP2=5.655  expZone2="[6.58           1]"  Rca=0.6  ti=2000  Dp=0  Neq0=0  Tsim=1e6  Ta1=25  Qeol=5.4*0.9  Reol=0.013333*1.2  Char_age=[2.3478, 3]  Dis_age=[2.3478, 10]  N1=1500  N2=10500  N3=1000  N4=1400  Ta2=45  N5=950
  Battery1 : spsBatteryLib/Battery  BatType=Lead-Acid  ShowTempParam=off  ThermalPreset="12.8V  40Ah  (LiFeMgPO4)"  ShowAgeParam=off  NomV=Vbat  NomQ=cap_bat  SOC=50  Batt_Tr=2  PresetModel=off  MaxQ=cap_bat  MinV=0.8*Vbat  FullV=1.1*Vbat  Dis_rate=Inom_bat  R=0.002  Normal_OP=0.9*cap_bat  expZone="[780   20]"  current=[250 500 750 1000]  Units=Ampere-hour  Tci=20  NomT=20  T2=-30  MaxQ2=4.8  FullV2=7.1  Normal_OP2=5.655  expZone2="[6.58           1]"  Rca=0.6  ti=2000  Dp=0  Neq0=0  Tsim=1e6  Ta1=25  Qeol=5.4*0.9  Reol=0.013333*1.2  Char_age=[2.3478, 3]  Dis_age=[2.3478, 10]  N1=1500  N2=10500  N3=1000  N4=1400  Ta2=45  N5=950
  Bus x : spsThreePhaseVIMeasurementLib/Three-Phase V-I Measurement  VoltageMeasurement=phase-to-ground  SetLabelV=off  LabelV=Vabc  Vpu=off  VpuLL=off  CurrentMeasurement=yes  SetLabelI=off  LabelI=Iabc  Ipu=off  Pbase=100e6  Vbase=13.8e3  OutputType=Complex  PhasorSimulation=off  PSBequivalent=0
  Cdc link : spsSeriesRLCBranchLib/Series RLC Branch  Commented=on  LConnTagsString=__new0  RConnTagsString=__new0  BranchType=C  Resistance=0.001  Inductance=1e-3  SetiL0=off  InitialCurrent=0  Capacitance=Cdc  Setx0=on  InitialVoltage=1500  Measurements=None
  Cdc link1 : spsSeriesRLCBranchLib/Series RLC Branch  LConnTagsString=__new0  RConnTagsString=__new0  BranchType=C  Resistance=0.001  Inductance=1e-3  SetiL0=off  InitialCurrent=0  Capacitance=Cdc  Setx0=on  InitialVoltage=1500  Measurements=None
  Current Measurement1 : spsCurrentMeasurementLib/Current Measurement  PhasorSimulation=off  OutputType=Complex  PSBequivalent=0
  Current Measurement2 : spsCurrentMeasurementLib/Current Measurement  Commented=on  PhasorSimulation=off  OutputType=Complex  PSBequivalent=0
  Current Measurement3 : spsCurrentMeasurementLib/Current Measurement  PhasorSimulation=off  OutputType=Complex  PSBequivalent=0
  DC-DC Converter Bidirectional1 : Subsystem
  DC-DC Converter Bidirectional2 : Subsystem  Commented=on
  DC-DC Converter Unidirectional : Subsystem  Commented=on
  DC-DC Converter Unidirectional1 : Subsystem
  From2 : From  Commented=on  GotoTag=Vdc
  Goto2 : Goto  Commented=on  GotoTag=Vdc
  Ground{1,3..5} (4 alike) : spsGroundLib/Ground  Commented=on  LConnTagsString=a
  Ground{2,9,12,14} (4 alike) : spsGroundLib/Ground  LConnTagsString=a
  Inverter : Subsystem
  Inverter1 : Subsystem  Commented=on
  Irradiance : Constant  Commented=on  Value=1000
  Irradiance1 : Constant  Value=1000
  Ldc link : spsSeriesRLCBranchLib/Series RLC Branch  Commented=on  LConnTagsString=__new0  RConnTagsString=__new0  BranchType=L  Resistance=0.002  Inductance=10e-3  SetiL0=off  InitialCurrent=0  Capacitance=5e-3  Setx0=on  InitialVoltage=0  Measurements=None
  Ldc1 : spsSeriesRLCBranchLib/Series RLC Branch  LConnTagsString=__new0  RConnTagsString=__new0  BranchType=L  Resistance=0.002  Inductance=10e-3  SetiL0=off  InitialCurrent=0  Capacitance=5e-3  Setx0=on  InitialVoltage=0  Measurements=None
  Low-Pass Filter (Discrete or Continuous) : eeGeneralControl/Low-Pass Filter (Discrete or Continuous)  Commented=on  K=1  T=1/(2*pi*5)  B=inf  A=-inf  init_option=Inherited from block input  x0=0  Ts=-1
  Low-Pass Filter (Discrete or Continuous)2 : eeGeneralControl/Low-Pass Filter (Discrete or Continuous)  Commented=on  K=1  T=1/(2*pi*5)  B=inf  A=-inf  init_option=Inherited from block input  x0=0  Ts=-1
  PV Solar Array : spsPVArrayLib/PV Array  Commented=on  Npar=278  Nser=15  PlotType=array @ 1000 W/m2 & specified temperatures  S_vec=[ 1000 800 500 300 100 ]  Temp_C_vec=[ 20 25 30 35 ]  ModuleName=Sunpower SPR-X22-480-COM  PlotWhenSelected=off  Pm=480.32  Ncell=128  Voc=92.9  Isc=6.48  Vm=79  Im=6.08  beta_Voc_pc=-0.293  alpha_Isc_pc=0.031003  beta_Voc=-0.2722  alpha_Isc=0.002009  IL=6.4884  I0=1.5908e-11  nI=1.0576  Rsh=598.2816  Rs=0.48607  RobustModel=off  RobustCellTemperature=313.3991  BAL=on  Tc=1e-6  Tfilter=5e-5
  PV Solar Array1 : spsPVArrayLib/PV Array  Npar=278  Nser=15  PlotType=array @ 1000 W/m2 & specified temperatures  S_vec=[ 1000 800 500 300 100 ]  Temp_C_vec=[ 20 25 30 35 ]  ModuleName=Sunpower SPR-X22-480-COM  PlotWhenSelected=off  Pm=480.32  Ncell=128  Voc=92.9  Isc=6.48  Vm=79  Im=6.08  beta_Voc_pc=-0.293  alpha_Isc_pc=0.031003  beta_Voc=-0.2722  alpha_Isc=0.002009  IL=6.4884  I0=1.5908e-11  nI=1.0576  Rsh=598.2816  Rs=0.48607  RobustModel=off  RobustCellTemperature=313.3991  BAL=on  Tc=1e-6  Tfilter=5e-5
  PV model2 : spsThreePhaseSourceLib/Three-Phase Source  InternalConnection=Yg  VoltagePhases=off  Voltage=(345000)*1  PhaseAngle=0  Voltage_phases=[25e3 25e3 25e3]/sqrt(3)  PhaseAngles_phases=[0 -120 +120]  Frequency=fg  NonIdealSource=off  SpecifyImpedance=off  Resistance=0.8929  Inductance=16.58e-3  ShortCircuitLevel=100e6  BaseVoltage=25e3  XRratio=7  BusType=swing  Pref=1993000  Qref=10680  Prefabc=[10e3, 10e3, 10e3]  Qrefabc=[0, 0, 0]  Qmin=-Inf  Qmax=Inf
  Power (Positive-Sequence) : spsPowerPositiveSequenceLib/Power (Positive-Sequence)  Commented=on  Freq=50  Vinit=[0, 0]  Iinit=[0, 0]  Ts=1e-5
      settings: LibrarySourceBlock=|
      | sps_lib/Sensors and Measurements/Power
      | (Positive-Sequence)
  Product : Product  Commented=on
  Scope3 : Scope  Commented=on  NumInputPorts=2
  Scope5 : Scope  Commented=on  NumInputPorts=2
  Scope9 : Scope  Commented=on  NumInputPorts=3
  Temp1 : Constant  Value=25
  Temperature : Constant  Commented=on  Value=25
  Three-Phase Transformer : spsThreePhaseTransformerTwoWindingsLib/Three-Phase Transformer (Two Windings)  Winding1Connection=Yg  Winding2Connection=Delta (D1)  CoreType=Three single-phase transformers  SetSaturation=off  Hysteresis=off  DataFile='hysteresis'  SetInitialFlux=off  Measurements=None  UNITS=pu  NominalPower=[ Pinv*2 , fg ]  Winding1=[Vbase 1e-6 1e-6]  Winding2=[Vac_inv 1e-6 1e-6]  Rm=500  Lm=1000  L0=0.5  Saturation=[0 0;0.01 0.9;0.05 1]  InitialFluxes=[-1.0025142026259 0.501432695325379 0.501081507300505]  BreakLoop=off  DiscreteSolver=Trapezoidal iterative  DataType=off  TransfoNumber=1
  Voltage Measurement1 : spsVoltageMeasurementLib/Voltage Measurement  PhasorSimulation=off  OutputType=Complex  PSBequivalent=0
  Voltage Measurement2 : spsVoltageMeasurementLib/Voltage Measurement  PhasorSimulation=off  OutputType=Complex  PSBequivalent=0
  Voltage Measurement3 : spsVoltageMeasurementLib/Voltage Measurement  Commented=on  PhasorSimulation=off  OutputType=Complex  PSBequivalent=0
  a : PMIOPort  Side=Right
  b : PMIOPort  Port=2  Side=Right
  c : PMIOPort  Port=3  Side=Right
  wires:
  Voltage Measurement2/1 -> Scope5/1  "Vout"
  Irradiance1/1 -> PV Solar Array1/1
  Low-Pass Filter (Discrete or Continuous)/1 -> Scope3/1  "Pout"
  Power (Positive-Sequence)/1 -> Low-Pass Filter (Discrete or Continuous)/1
  Current Measurement1/1 -> Scope5/2  "iout"
  Voltage Measurement1/1 -> [Vdc], Product/1, Scope9/1
  Current Measurement3/1 -> Product/2, Scope9/2
  Low-Pass Filter (Discrete or Continuous)2/1 -> Scope3/2  "Qout"
  [Vdc] -> DC-DC Converter Bidirectional1/1(Vdclink)
  Bus x/2 -> Power (Positive-Sequence)/2
  Temp1/1 -> PV Solar Array1/2
  Bus x/1 -> Power (Positive-Sequence)/1
  Power (Positive-Sequence)/2 -> Low-Pass Filter (Discrete or Continuous)2/1
  Product/1 -> Scope9/3
  Temperature/1 -> PV Solar Array/2
  Voltage Measurement3/1 -> Goto2/1
  From2/1 -> DC-DC Converter Bidirectional2/1(Vdclink)
  Irradiance/1 -> PV Solar Array/1
  connections:
  Inverter/RConn1 -- Current Measurement1/LConn1
  PV Solar Array1/RConn1 -- DC-DC Converter Unidirectional1/LConn1
  Voltage Measurement2/LConn1 -- Current Measurement1/RConn1 -- Three-Phase Transformer/RConn1
  Voltage Measurement2/LConn2 -- Inverter/RConn2 -- Three-Phase Transformer/RConn2
  Inverter/LConn1 -- Voltage Measurement1/LConn1 -- Current Measurement3/RConn1
  Three-Phase Transformer/RConn3 -- Inverter/RConn3
  Battery1/LConn2 -- Ground2/LConn1
  Three-Phase Transformer/LConn3 -- Bus x/LConn3
  Voltage Measurement1/LConn2 -- Ground9/LConn1
  PV Solar Array1/RConn2 -- Ground14/LConn1
  Battery1/LConn1 -- DC-DC Converter Bidirectional1/LConn1
  Ground12/LConn1 -- Cdc link1/RConn1
  Three-Phase Transformer/LConn1 -- Bus x/LConn1
  Current Measurement3/LConn1 -- Cdc link1/LConn1 -- DC-DC Converter Bidirectional1/RConn1 -- Ldc1/RConn1
  Three-Phase Transformer/LConn2 -- Bus x/LConn2
  Ldc1/LConn1 -- DC-DC Converter Unidirectional1/RConn1
  Bus x/RConn2 -- b/RConn1 -- PV model2/RConn2
  Bus x/RConn1 -- a/RConn1 -- PV model2/RConn1
  Bus x/RConn3 -- c/RConn1 -- PV model2/RConn3
  Ldc link/RConn1 -- Cdc link/LConn1 -- Current Measurement2/LConn1 -- Voltage Measurement3/LConn1 -- DC-DC Converter Bidirectional2/RConn1
  Ldc link/LConn1 -- DC-DC Converter Unidirectional/RConn1
  PV Solar Array/RConn1 -- DC-DC Converter Unidirectional/LConn1
  PV Solar Array/RConn2 -- Ground3/LConn1
  Voltage Measurement3/LConn2 -- Ground5/LConn1
  Ground1/LConn1 -- Cdc link/RConn1
  Battery/LConn2 -- Ground4/LConn1
  Battery/LConn1 -- DC-DC Converter Bidirectional2/LConn1

== system V2G_FDCC/PV system4 ==
  note: P = 1.96e6
      | Q = -0.6842
  Battery1 : spsBatteryLib/Battery  BatType=Lead-Acid  ShowTempParam=off  ThermalPreset="12.8V  40Ah  (LiFeMgPO4)"  ShowAgeParam=off  NomV=Vbat  NomQ=cap_bat  SOC=50  Batt_Tr=2  PresetModel=off  MaxQ=cap_bat  MinV=0.8*Vbat  FullV=1.1*Vbat  Dis_rate=Inom_bat  R=0.002  Normal_OP=0.9*cap_bat  expZone="[780   20]"  current=[250 500 750 1000]  Units=Ampere-hour  Tci=20  NomT=20  T2=-30  MaxQ2=4.8  FullV2=7.1  Normal_OP2=5.655  expZone2="[6.58           1]"  Rca=0.6  ti=2000  Dp=0  Neq0=0  Tsim=1e6  Ta1=25  Qeol=5.4*0.9  Reol=0.013333*1.2  Char_age=[2.3478, 3]  Dis_age=[2.3478, 10]  N1=1500  N2=10500  N3=1000  N4=1400  Ta2=45  N5=950
  Bus x : spsThreePhaseVIMeasurementLib/Three-Phase V-I Measurement  VoltageMeasurement=phase-to-ground  SetLabelV=off  LabelV=Vabc  Vpu=off  VpuLL=off  CurrentMeasurement=yes  SetLabelI=off  LabelI=Iabc  Ipu=off  Pbase=100e6  Vbase=13.8e3  OutputType=Complex  PhasorSimulation=off  PSBequivalent=0
  Cdc link1 : spsSeriesRLCBranchLib/Series RLC Branch  LConnTagsString=__new0  RConnTagsString=__new0  BranchType=C  Resistance=0.001  Inductance=1e-3  SetiL0=off  InitialCurrent=0  Capacitance=Cdc  Setx0=on  InitialVoltage=1500  Measurements=None
  Current Measurement1 : spsCurrentMeasurementLib/Current Measurement  PhasorSimulation=off  OutputType=Complex  PSBequivalent=0
  Current Measurement3 : spsCurrentMeasurementLib/Current Measurement  PhasorSimulation=off  OutputType=Complex  PSBequivalent=0
  DC-DC Converter Bidirectional1 : Subsystem
  DC-DC Converter Unidirectional1 : Subsystem
  Ground{2,9,12,14} (4 alike) : spsGroundLib/Ground  LConnTagsString=a
  Inverter : Subsystem
  Irradiance1 : Constant  Value=1000
  Ldc1 : spsSeriesRLCBranchLib/Series RLC Branch  LConnTagsString=__new0  RConnTagsString=__new0  BranchType=L  Resistance=0.002  Inductance=10e-3  SetiL0=off  InitialCurrent=0  Capacitance=5e-3  Setx0=on  InitialVoltage=0  Measurements=None
  Low-Pass Filter (Discrete or Continuous) : eeGeneralControl/Low-Pass Filter (Discrete or Continuous)  Commented=on  K=1  T=1/(2*pi*5)  B=inf  A=-inf  init_option=Inherited from block input  x0=0  Ts=-1
  Low-Pass Filter (Discrete or Continuous)2 : eeGeneralControl/Low-Pass Filter (Discrete or Continuous)  Commented=on  K=1  T=1/(2*pi*5)  B=inf  A=-inf  init_option=Inherited from block input  x0=0  Ts=-1
  PV Solar Array1 : spsPVArrayLib/PV Array  Npar=278  Nser=15  PlotType=array @ 1000 W/m2 & specified temperatures  S_vec=[ 1000 800 500 300 100 ]  Temp_C_vec=[ 20 25 30 35 ]  ModuleName=Sunpower SPR-X22-480-COM  PlotWhenSelected=off  Pm=480.32  Ncell=128  Voc=92.9  Isc=6.48  Vm=79  Im=6.08  beta_Voc_pc=-0.293  alpha_Isc_pc=0.031003  beta_Voc=-0.2722  alpha_Isc=0.002009  IL=6.4884  I0=1.5908e-11  nI=1.0576  Rsh=598.2816  Rs=0.48607  RobustModel=off  RobustCellTemperature=313.3991  BAL=on  Tc=1e-6  Tfilter=5e-5
  PV model2 : spsThreePhaseSourceLib/Three-Phase Source  Commented=on  InternalConnection=Yg  VoltagePhases=off  Voltage=(345000)*1  PhaseAngle=0  Voltage_phases=[25e3 25e3 25e3]/sqrt(3)  PhaseAngles_phases=[0 -120 +120]  Frequency=fg  NonIdealSource=off  SpecifyImpedance=off  Resistance=0.8929  Inductance=16.58e-3  ShortCircuitLevel=100e6  BaseVoltage=25e3  XRratio=7  BusType=swing  Pref=1993000  Qref=10680  Prefabc=[10e3, 10e3, 10e3]  Qrefabc=[0, 0, 0]  Qmin=-Inf  Qmax=Inf
  Power (Positive-Sequence) : spsPowerPositiveSequenceLib/Power (Positive-Sequence)  Commented=on  Freq=50  Vinit=[0, 0]  Iinit=[0, 0]  Ts=1e-5
      settings: LibrarySourceBlock=|
      | sps_lib/Sensors and Measurements/Power
      | (Positive-Sequence)
  Product : Product  Commented=on
  Scope3 : Scope  Commented=on  NumInputPorts=2
  Scope5 : Scope  Commented=on  NumInputPorts=2
  Scope9 : Scope  Commented=on  NumInputPorts=3
  Temp1 : Constant  Value=25
  Three-Phase Transformer : spsThreePhaseTransformerTwoWindingsLib/Three-Phase Transformer (Two Windings)  Winding1Connection=Yg  Winding2Connection=Delta (D1)  CoreType=Three single-phase transformers  SetSaturation=off  Hysteresis=off  DataFile='hysteresis'  SetInitialFlux=off  Measurements=None  UNITS=pu  NominalPower=[ Pinv*2 , fg ]  Winding1=[Vbase 1e-6 1e-6]  Winding2=[Vac_inv 1e-6 1e-6]  Rm=500  Lm=1000  L0=0.5  Saturation=[0 0;0.01 0.9;0.05 1]  InitialFluxes=[-1.0025142026259 0.501432695325379 0.501081507300505]  BreakLoop=off  DiscreteSolver=Trapezoidal iterative  DataType=off  TransfoNumber=1
  Voltage Measurement1 : spsVoltageMeasurementLib/Voltage Measurement  PhasorSimulation=off  OutputType=Complex  PSBequivalent=0
  Voltage Measurement2 : spsVoltageMeasurementLib/Voltage Measurement  PhasorSimulation=off  OutputType=Complex  PSBequivalent=0
  a : PMIOPort  Side=Right
  b : PMIOPort  Port=2  Side=Right
  c : PMIOPort  Port=3  Side=Right
  wires:
  Voltage Measurement2/1 -> Scope5/1  "Vout"
  Irradiance1/1 -> PV Solar Array1/1
  Low-Pass Filter (Discrete or Continuous)/1 -> Scope3/1  "Pout"
  Power (Positive-Sequence)/1 -> Low-Pass Filter (Discrete or Continuous)/1
  Current Measurement1/1 -> Scope5/2  "iout"
  Voltage Measurement1/1 -> [Vdc], Product/1, Scope9/1
  Current Measurement3/1 -> Product/2, Scope9/2
  Low-Pass Filter (Discrete or Continuous)2/1 -> Scope3/2  "Qout"
  [Vdc] -> DC-DC Converter Bidirectional1/1(Vdclink)
  Bus x/2 -> Power (Positive-Sequence)/2
  Temp1/1 -> PV Solar Array1/2
  Bus x/1 -> Power (Positive-Sequence)/1
  Power (Positive-Sequence)/2 -> Low-Pass Filter (Discrete or Continuous)2/1
  Product/1 -> Scope9/3
  connections:
  Inverter/RConn1 -- Current Measurement1/LConn1
  PV Solar Array1/RConn1 -- DC-DC Converter Unidirectional1/LConn1
  Voltage Measurement2/LConn1 -- Current Measurement1/RConn1 -- Three-Phase Transformer/RConn1
  Voltage Measurement2/LConn2 -- Inverter/RConn2 -- Three-Phase Transformer/RConn2
  Inverter/LConn1 -- Voltage Measurement1/LConn1 -- Current Measurement3/RConn1
  Three-Phase Transformer/RConn3 -- Inverter/RConn3
  Battery1/LConn2 -- Ground2/LConn1
  Three-Phase Transformer/LConn3 -- Bus x/LConn3
  Voltage Measurement1/LConn2 -- Ground9/LConn1
  PV Solar Array1/RConn2 -- Ground14/LConn1
  Battery1/LConn1 -- DC-DC Converter Bidirectional1/LConn1
  Ground12/LConn1 -- Cdc link1/RConn1
  Three-Phase Transformer/LConn1 -- Bus x/LConn1
  Current Measurement3/LConn1 -- Cdc link1/LConn1 -- DC-DC Converter Bidirectional1/RConn1 -- Ldc1/RConn1
  Three-Phase Transformer/LConn2 -- Bus x/LConn2
  Ldc1/LConn1 -- DC-DC Converter Unidirectional1/RConn1
  Bus x/RConn2 -- b/RConn1 -- PV model2/RConn2
  Bus x/RConn1 -- a/RConn1 -- PV model2/RConn1
  Bus x/RConn3 -- c/RConn1 -- PV model2/RConn3

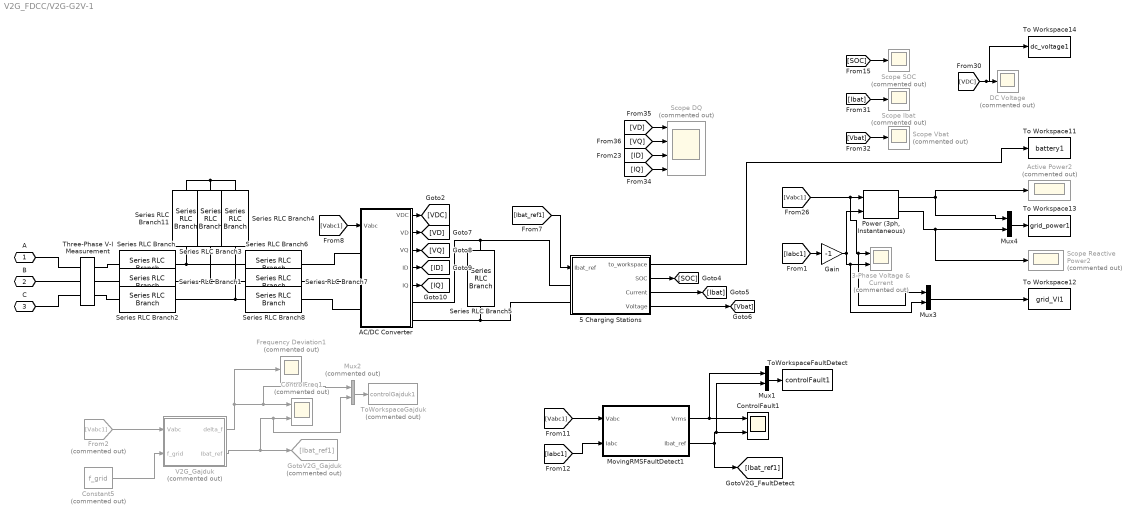
== system V2G_FDCC/V2G-G2V-1 ==
  3-Phase Voltage & Current : Scope  Commented=on  NumInputPorts=2
  5 Charging Stations : Subsystem
  AC/DC Converter : Subsystem
  Active Power2 : Scope  Commented=on
  Constant5 : Constant  Commented=on  Value=f_grid
  ControlFault1 : Scope  NumInputPorts=2
  ControlFreq1 : Scope  Commented=on  NumInputPorts=2
  DC Voltage : Scope  Commented=on
  Frequency Deviation1 : Scope  Commented=on
  From2 : From  Commented=on  GotoTag=Vabc1  TagVisibility=global
  Gain : Gain  Gain=-1
  GotoV2G_Gajduk : Goto  Commented=on  GotoTag=Ibat_ref1
  MovingRMSFaultDetect1 : Subsystem
  Mux1 : Mux  Inputs=2
  Mux2 : Mux  Commented=on  Inputs=2
  Mux3 : Mux  Inputs=2
  Mux4 : Mux  Inputs=2
  "Power (3ph, Instantaneous)" : spsPower3phInstantaneousLib/Power (3ph, Instantaneous)
  Scope DQ : Scope  Commented=on  NumInputPorts=4
  Scope Ibat : Scope  Commented=on
  Scope Reactive Power2 : Scope  Commented=on
  Scope SOC : Scope  Commented=on
  Scope Vbat : Scope  Commented=on
  Series RLC Branch : spsSeriesRLCBranchLib/Series RLC Branch  LConnTagsString=__new0  RConnTagsString=__new0  BranchType=L  Resistance=1  Inductance=Lgrid  SetiL0=off  InitialCurrent=0  Capacitance=1e-6  Setx0=off  InitialVoltage=0  Measurements=None
  Series RLC Branch1 : spsSeriesRLCBranchLib/Series RLC Branch  LConnTagsString=__new0  RConnTagsString=__new0  BranchType=L  Resistance=1  Inductance=Lgrid  SetiL0=off  InitialCurrent=0  Capacitance=1e-6  Setx0=off  InitialVoltage=0  Measurements=None
  Series RLC Branch11 : spsSeriesRLCBranchLib/Series RLC Branch  LConnTagsString=__new0  RConnTagsString=__new0  BranchType=RC  Resistance=Rd  Inductance=Lbuckboost  SetiL0=off  InitialCurrent=0  Capacitance=Cf  Setx0=off  InitialVoltage=0  Measurements=None
  Series RLC Branch2 : spsSeriesRLCBranchLib/Series RLC Branch  LConnTagsString=__new0  RConnTagsString=__new0  BranchType=L  Resistance=1  Inductance=Lgrid  SetiL0=off  InitialCurrent=0  Capacitance=1e-6  Setx0=off  InitialVoltage=0  Measurements=None
  Series RLC Branch3 : spsSeriesRLCBranchLib/Series RLC Branch  LConnTagsString=__new0  RConnTagsString=__new0  BranchType=RC  Resistance=Rd  Inductance=Lbuckboost  SetiL0=off  InitialCurrent=0  Capacitance=Cf  Setx0=off  InitialVoltage=0  Measurements=None
  Series RLC Branch4 : spsSeriesRLCBranchLib/Series RLC Branch  LConnTagsString=__new0  RConnTagsString=__new0  BranchType=RC  Resistance=Rd  Inductance=Lbuckboost  SetiL0=off  InitialCurrent=0  Capacitance=Cf  Setx0=off  InitialVoltage=0  Measurements=None
  Series RLC Branch5 : spsSeriesRLCBranchLib/Series RLC Branch  LConnTagsString=__new0  RConnTagsString=__new0  BranchType=C  Resistance=R_Vdc  Inductance=1e-3  SetiL0=off  InitialCurrent=0  Capacitance=C_Vdc  Setx0=on  InitialVoltage=V0_Vdc  Measurements=None
  Series RLC Branch6 : spsSeriesRLCBranchLib/Series RLC Branch  LConnTagsString=__new0  RConnTagsString=__new0  BranchType=L  Resistance=1  Inductance=Linv  SetiL0=off  InitialCurrent=0  Capacitance=1e-6  Setx0=off  InitialVoltage=0  Measurements=None
  Series RLC Branch7 : spsSeriesRLCBranchLib/Series RLC Branch  LConnTagsString=__new0  RConnTagsString=__new0  BranchType=L  Resistance=1  Inductance=Linv  SetiL0=off  InitialCurrent=0  Capacitance=1e-6  Setx0=off  InitialVoltage=0  Measurements=None
  Series RLC Branch8 : spsSeriesRLCBranchLib/Series RLC Branch  LConnTagsString=__new0  RConnTagsString=__new0  BranchType=L  Resistance=1  Inductance=Linv  SetiL0=off  InitialCurrent=0  Capacitance=1e-6  Setx0=off  InitialVoltage=0  Measurements=None
  Three-Phase V-I Measurement : spsThreePhaseVIMeasurementLib/Three-Phase V-I Measurement  VoltageMeasurement=phase-to-ground  SetLabelV=on  LabelV=Vabc1  Vpu=off  VpuLL=off  CurrentMeasurement=yes  SetLabelI=on  LabelI=Iabc1  Ipu=off  Pbase=100e6  Vbase=500e3  OutputType=Complex  PhasorSimulation=off  PSBequivalent=0
  To Workspace11 : ToWorkspace  VariableName=battery1  SaveFormat=Timeseries  SampleTime=-1
  To Workspace12 : ToWorkspace  VariableName=grid_VI1  SaveFormat=Timeseries  SampleTime=-1
  To Workspace13 : ToWorkspace  VariableName=grid_power1  SaveFormat=Timeseries  SampleTime=-1
  To Workspace14 : ToWorkspace  VariableName=dc_voltage1  SaveFormat=Timeseries  SampleTime=-1
  ToWorkspaceFaultDetect : ToWorkspace  VariableName=controlFault1  SaveFormat=Timeseries  SampleTime=-1
  ToWorkspaceGajduk : ToWorkspace  Commented=on  VariableName=controlGajduk1  SaveFormat=Timeseries  SampleTime=-1
  V2G_Gajduk : Subsystem  Commented=on
  A : PMIOPort  Side=Left
  B : PMIOPort  Port=2  Side=Left
  C : PMIOPort  Port=3  Side=Left
  wires:
  AC/DC Converter/3(VQ) -> [VQ]
  [Iabc1] -> Gain/1
  [ID] -> Scope DQ/3
  AC/DC Converter/1(VDC) -> [VDC]
  AC/DC Converter/4(ID) -> [ID]
  [Ibat] -> Scope Ibat/1
  Gain/1 -> Mux3/2, 3-Phase Voltage & Current/2, "Power (3ph, Instantaneous)"/2
  AC/DC Converter/2(VD) -> [VD]
  [IQ] -> Scope DQ/4
  [VD] -> Scope DQ/1
  [VQ] -> Scope DQ/2
  [Ibat_ref1] -> 5 Charging Stations/1(Ibat_ref)
  5 Charging Stations/2(SOC) -> [SOC]
  5 Charging Stations/3(Current) -> [Ibat]
  [Vbat] -> Scope Vbat/1
  5 Charging Stations/4(Voltage) -> [Vbat]
  [Vabc1] -> Mux3/1, 3-Phase Voltage & Current/1, "Power (3ph, Instantaneous)"/1
  AC/DC Converter/5(IQ) -> [IQ]
  [Vabc1] -> AC/DC Converter/1(Vabc)
  [SOC] -> Scope SOC/1
  Mux4/1 -> To Workspace13/1
  "Power (3ph, Instantaneous)"/2 -> Scope Reactive Power2/1, Mux4/2
  [VDC] -> To Workspace14/1, DC Voltage/1
  Mux3/1 -> To Workspace12/1
  "Power (3ph, Instantaneous)"/1 -> Mux4/1, Active Power2/1
  5 Charging Stations/1(to_workspace) -> To Workspace11/1
  V2G_Gajduk/2(Ibat_ref) -> Mux2/2, ControlFreq1/2, GotoV2G_Gajduk/1
  V2G_Gajduk/1(delta_f) -> Mux2/1, ControlFreq1/1, Frequency Deviation1/1
  Constant5/1 -> V2G_Gajduk/2(f_grid)
  Mux2/1 -> ToWorkspaceGajduk/1
  From2/1 -> V2G_Gajduk/1(Vabc)
  Mux1/1 -> ToWorkspaceFaultDetect/1
  [Iabc1] -> MovingRMSFaultDetect1/2(Iabc)
  MovingRMSFaultDetect1/1(Vrms) -> Mux1/1, ControlFault1/1
  [Vabc1] -> MovingRMSFaultDetect1/1(Vabc)
  MovingRMSFaultDetect1/2(Ibat_ref) -> Mux1/2, ControlFault1/2, [Ibat_ref1]
  connections:
  Series RLC Branch5/LConn1 -- 5 Charging Stations/LConn1 -- AC/DC Converter/RConn1
  Series RLC Branch6/LConn1 -- Series RLC Branch11/LConn1 -- Series RLC Branch/RConn1
  Series RLC Branch4/LConn1 -- Series RLC Branch8/LConn1 -- Series RLC Branch2/RConn1
  B/RConn1 -- Three-Phase V-I Measurement/LConn2
  Series RLC Branch/LConn1 -- Three-Phase V-I Measurement/RConn1
  A/RConn1 -- Three-Phase V-I Measurement/LConn1
  AC/DC Converter/LConn1 -- Series RLC Branch6/RConn1
  AC/DC Converter/LConn3 -- Series RLC Branch8/RConn1
  Series RLC Branch3/LConn1 -- Series RLC Branch1/RConn1 -- Series RLC Branch7/LConn1
  Series RLC Branch1/LConn1 -- Three-Phase V-I Measurement/RConn2
  5 Charging Stations/LConn2 -- Series RLC Branch5/RConn1 -- AC/DC Converter/RConn2
  Series RLC Branch11/RConn1 -- Series RLC Branch4/RConn1 -- Series RLC Branch3/RConn1
  C/RConn1 -- Three-Phase V-I Measurement/LConn3
  AC/DC Converter/LConn2 -- Series RLC Branch7/RConn1
  Series RLC Branch2/LConn1 -- Three-Phase V-I Measurement/RConn3
